simulink model "PSO_ZVD"  (R2021a)
settings: Solver=VariableStepAuto  StartTime=0.0  StopTime=20  RelTol=1e-3
InitFcn:
  | ml=2;
  | 
  | mc=0.5;
  | M2=0.5;
  | 
  | mt=5;
  | g=9.81;
  | l_ref=0.1;
  | l_ini=1;
  | l=l_ini;
  | x_ref=1;
  | n1=5;n2=1;
  | 
  | %ADRC' s parameter caculation
  | %b0 = (ml+mc)/(mc*ml +mc*mt+ml*mt); %Hieu
  | b0=(ml+mc)/(mt*mc+2*ml*mc+mt*ml+ml^2+mc^2); %Enhanced-coupling
  | k_ESO = 100;
  | T_set  = 6;
  | 
  | s_cl = -5.85/T_set;
  | Kp   = s_cl^2;
  | Kd   = -2*s_cl;
  | 
  | s_ESO = k_ESO*s_cl;
  | l1        = -3*s_ESO;
  | l2        = 3*( s_ESO)^2;
  | l3        = -(s_ESO)^3;
  | 
  | %b1 = (mt+mc)/(mc*ml +mc*mt+ml*mt);
  | b1=1/(ml+mc);
  | k_ESO1 =100;
  | T_set1  = 3;
  | s_cl1 = -5.85/T_set1;
  | Kp1   = s_cl1^2;
  | Kd1   = -2*s_cl1;
  | 
  | s_ESO1 = k_ESO1*s_cl1;
  | l11        = -3*s_ESO1;
  | l21        = 3*( s_ESO1)^2;
  | l31        = -(s_ESO1)^3;
  | 
  | 
  | L1=l_ini;
  | %L2=0.5;
  | L2=0.1;
  | m1=2;
  | m2=mc;
  | m=5;
  | %Bo input shaping
  | alpha = (1/L1 + 1/L2)*(m1+M2)/m1;
  | beta = (((m1+M2)/m1)^2)*((1/L1 + 1/L2)^2) - 4*(m1+M2)/(m1*L1*L2);
  | w1 = sqrt(g*(alpha - sqrt(beta))/2);
  | w2 = sqrt(g*(alpha + sqrt(beta))/2);
  | damping_ratio = 0;
  | wd1 = w1*sqrt(1-damping_ratio^2);
  | wd2 = w2*sqrt(1-damping_ratio^2);
  | k = exp(damping_ratio*pi/sqrt(1-damping_ratio^2));
  | 
  | %ZVD1
  | t1_ZVD_1=pi/wd1;
  | ... (+27 lines)
values from neighbouring files (symbols this model uses):
  particle = repmat(empty_particle, nPop, 1)    [PSO16_12.m]    (also in PSO_ZVD.m)
undefined symbols (not defined in the file or in its folder): i, li, xi
libraries: neural x101, simulink_extras x13, simulink x3
(part 3 of 34)

== system PSO_ZVD/RBF_ET4_m=5_m1=2/ADRC 6 ==
  ref : Inport
  x : Inport  Port=2
  Gain : Gain  Gain=Kp1
  Gain1 : Gain  Gain=Kd1
  Gain2 : Gain  Gain=1/b1
  Observer : Subsystem
  Sum : Sum  Inputs=|+-
  Sum3 : Sum  Inputs=|+-
  Sum4 : Sum  Inputs=|+-
  u : Outport
  wires:
  Sum4/1 -> Gain2/1
  Sum/1 -> Gain/1
  Gain2/1 -> u/1, Observer/1(u)
  x/1 -> Observer/2(x)
  Sum3/1 -> Sum4/1
  Observer/2(x2) -> Gain1/1
  Gain1/1 -> Sum3/2
  Gain/1 -> Sum3/1
  ref/1 -> Sum/1
  Observer/1(x3) -> Sum4/2
  Observer/3(x1) -> Sum/2

== system PSO_ZVD/RBF_ET4_m=5_m1=2/ADRC 7 ==
  ref : Inport
  x : Inport  Port=2
  Gain : Gain  Gain=Kp
  Gain1 : Gain  Gain=Kd
  Gain2 : Gain  Gain=1/b0
  Observer : Subsystem
  Sum : Sum  Inputs=|+-
  Sum3 : Sum  Inputs=|+-
  Sum4 : Sum  Inputs=|+-
  u : Outport
  wires:
  Sum4/1 -> Gain2/1
  Sum/1 -> Gain/1
  Gain2/1 -> u/1, Observer/1(u)
  x/1 -> Observer/2(x)
  Sum3/1 -> Sum4/1
  Observer/2(x2) -> Gain1/1
  Gain1/1 -> Sum3/2
  Gain/1 -> Sum3/1
  ref/1 -> Sum/1
  Observer/1(x3) -> Sum4/2
  Observer/3(x1) -> Sum/2

== system PSO_ZVD/RBF_ET4_m=5_m1=2/ADRC 8 ==
  ref : Inport
  x : Inport  Port=2
  Gain : Gain  Gain=Kp1
  Gain1 : Gain  Gain=Kd1
  Gain2 : Gain  Gain=1/b1
  Observer : Subsystem
  Sum : Sum  Inputs=|+-
  Sum3 : Sum  Inputs=|+-
  Sum4 : Sum  Inputs=|+-
  u : Outport
  wires:
  Sum4/1 -> Gain2/1
  Sum/1 -> Gain/1
  Gain2/1 -> u/1, Observer/1(u)
  x/1 -> Observer/2(x)
  Sum3/1 -> Sum4/1
  Observer/2(x2) -> Gain1/1
  Gain1/1 -> Sum3/2
  Gain/1 -> Sum3/1
  ref/1 -> Sum/1
  Observer/1(x3) -> Sum4/2
  Observer/3(x1) -> Sum/2

== system PSO_ZVD/RBF_ET4_m=5_m1=2/ADRC 9 ==
  ref : Inport
  x : Inport  Port=2
  Gain : Gain  Gain=Kp
  Gain1 : Gain  Gain=Kd
  Gain2 : Gain  Gain=1/b0
  Observer : Subsystem
  Sum : Sum  Inputs=|+-
  Sum3 : Sum  Inputs=|+-
  Sum4 : Sum  Inputs=|+-
  u : Outport
  wires:
  Sum4/1 -> Gain2/1
  Sum/1 -> Gain/1
  Gain2/1 -> u/1, Observer/1(u)
  x/1 -> Observer/2(x)
  Sum3/1 -> Sum4/1
  Observer/2(x2) -> Gain1/1
  Gain1/1 -> Sum3/2
  Gain/1 -> Sum3/1
  ref/1 -> Sum/1
  Observer/1(x3) -> Sum4/2
  Observer/3(x1) -> Sum/2

== system PSO_ZVD/RBF_ET4_m=5_m1=2/ETM1 ==
  In1 : Inport
  Gain : Gain  Gain=A1_etm4_2
  Gain1 : Gain  Gain=A2_etm4_2
  Gain2 : Gain  Gain=A3_etm4_2
  Gain3 : Gain  Gain=A4_etm4_2
  Sum : Sum  Inputs=++++
  Transport Delay : TransportDelay  DelayTime=t1_etm4_2
  Transport Delay1 : TransportDelay  DelayTime=t2_etm4_2
  Transport Delay2 : TransportDelay  DelayTime=t3_etm4_2
  ref : Outport
  wires:
  In1/1 -> Gain1/1, Gain3/1, Gain2/1, Gain/1
  Gain1/1 -> Transport Delay/1
  Transport Delay/1 -> Sum/2
  Sum/1 -> ref/1
  Gain2/1 -> Transport Delay1/1
  Gain/1 -> Sum/1
  Transport Delay1/1 -> Sum/3
  Gain3/1 -> Transport Delay2/1
  Transport Delay2/1 -> Sum/4

== system PSO_ZVD/RBF_ET4_m=5_m1=2/ETM2 ==
  ref_ETm4 : Inport
  ETM1 : Subsystem
  ETM4 : Subsystem
  ref1 : Scope
  ref2 : Scope
  ref3 : Scope
  ref_ETM4 : Outport
  wires:
  ETM1/1(Out1) -> ref2/1, ETM4/1(In1)  "ref_ZV"
  ETM4/1(Out1) -> ref3/1, ref_ETM4/1  "ref_ZV"
  ref_ETm4/1 -> ref1/1, ETM1/1(In1)

== system PSO_ZVD/RBF_ET4_m=5_m1=2/ETM3 ==
  In1 : Inport
  Gain : Gain  Gain=A1_etm4_1
  Gain1 : Gain  Gain=A2_etm4_1
  Gain2 : Gain  Gain=A3_etm4_1
  Gain3 : Gain  Gain=A4_etm4_1
  Sum : Sum  Inputs=++++
  Transport Delay : TransportDelay  DelayTime=t1_etm4_1
  Transport Delay1 : TransportDelay  DelayTime=t2_etm4_1
  Transport Delay2 : TransportDelay  DelayTime=t3_etm4_1
  ref : Outport
  wires:
  In1/1 -> Gain1/1, Gain3/1, Gain2/1, Gain/1
  Gain1/1 -> Transport Delay/1
  Transport Delay/1 -> Sum/2
  Sum/1 -> ref/1
  Gain2/1 -> Transport Delay1/1
  Gain/1 -> Sum/1
  Transport Delay1/1 -> Sum/3
  Gain3/1 -> Transport Delay2/1
  Transport Delay2/1 -> Sum/4

== system PSO_ZVD/RBF_ET4_m=5_m1=2/ETM4 ==
  In1 : Inport
  Gain : Gain  Gain=A1_etm4_2
  Gain1 : Gain  Gain=A2_etm4_2
  Gain2 : Gain  Gain=A3_etm4_2
  Gain3 : Gain  Gain=A4_etm4_2
  Sum : Sum  Inputs=++++
  Transport Delay : TransportDelay  DelayTime=t1_etm4_2
  Transport Delay1 : TransportDelay  DelayTime=t2_etm4_2
  Transport Delay2 : TransportDelay  DelayTime=t3_etm4_2
  ref : Outport
  wires:
  In1/1 -> Gain1/1, Gain3/1, Gain2/1, Gain/1
  Gain1/1 -> Transport Delay/1
  Transport Delay/1 -> Sum/2
  Sum/1 -> ref/1
  Gain2/1 -> Transport Delay1/1
  Gain/1 -> Sum/1
  Transport Delay1/1 -> Sum/3
  Gain3/1 -> Transport Delay2/1
  Transport Delay2/1 -> Sum/4

== system PSO_ZVD/RBF_ET4_m=5_m1=2/PSO-ETM1 ==
  In1 : Inport
  Input : Inport  Port=2
  Input1 : Inport  Port=3
  Input2 : Inport  Port=4
  Gain : Gain  Gain=0.1667
  Gain1 : Gain  Gain=0.3333
  Gain2 : Gain  Gain=0.3333
  Gain3 : Gain  Gain=0.1667
  Sum : Sum  Inputs=++++
  Variable Transport Delay : VariableTransportDelay  VariableDelayType=Variable transport delay  MaximumDelay=10
  Variable Transport Delay1 : VariableTransportDelay  VariableDelayType=Variable transport delay  MaximumDelay=10
  Variable Transport Delay2 : VariableTransportDelay  VariableDelayType=Variable transport delay  MaximumDelay=10
  Out1 : Outport
  wires:
  In1/1 -> Gain1/1, Gain3/1, Gain2/1, Gain/1
  Gain1/1 -> Variable Transport Delay/1
  Variable Transport Delay/1 -> Sum/2
  Sum/1 -> Out1/1
  Gain2/1 -> Variable Transport Delay1/1
  Gain/1 -> Sum/1
  Variable Transport Delay1/1 -> Sum/3
  Gain3/1 -> Variable Transport Delay2/1
  Variable Transport Delay2/1 -> Sum/4
  Input/1 -> Variable Transport Delay/2
  Input1/1 -> Variable Transport Delay1/2
  Input2/1 -> Variable Transport Delay2/2

== system PSO_ZVD/RBF_ET4_m=5_m1=2/PSO-ETM3 ==
  In1 : Inport
  Input : Inport  Port=2
  Input1 : Inport  Port=3
  Input2 : Inport  Port=4
  Gain : Gain  Gain=0.1667
  Gain1 : Gain  Gain=0.3333
  Gain2 : Gain  Gain=0.3333
  Gain3 : Gain  Gain=0.1667
  Sum : Sum  Inputs=++++
  Variable Transport Delay : VariableTransportDelay  VariableDelayType=Variable transport delay  MaximumDelay=10
  Variable Transport Delay1 : VariableTransportDelay  VariableDelayType=Variable transport delay  MaximumDelay=10
  Variable Transport Delay2 : VariableTransportDelay  VariableDelayType=Variable transport delay  MaximumDelay=10
  ref : Outport
  wires:
  In1/1 -> Gain1/1, Gain3/1, Gain2/1, Gain/1
  Gain1/1 -> Variable Transport Delay/1
  Variable Transport Delay/1 -> Sum/2
  Sum/1 -> ref/1
  Gain2/1 -> Variable Transport Delay1/1
  Gain/1 -> Sum/1
  Variable Transport Delay1/1 -> Sum/3
  Gain3/1 -> Variable Transport Delay2/1
  Variable Transport Delay2/1 -> Sum/4
  Input/1 -> Variable Transport Delay/2
  Input1/1 -> Variable Transport Delay1/2
  Input2/1 -> Variable Transport Delay2/2

== system PSO_ZVD/RBF_ET4_m=5_m1=2/PSO-ETM4 ==
  In1 : Inport
  Input : Inport  Port=2
  Input1 : Inport  Port=3
  Input2 : Inport  Port=4
  Gain : Gain  Gain=0.1667
  Gain1 : Gain  Gain=0.3333
  Gain2 : Gain  Gain=0.3333
  Gain3 : Gain  Gain=0.1667
  Sum : Sum  Inputs=++++
  Variable Transport Delay : VariableTransportDelay  VariableDelayType=Variable transport delay  MaximumDelay=10
  Variable Transport Delay1 : VariableTransportDelay  VariableDelayType=Variable transport delay  MaximumDelay=10
  Variable Transport Delay2 : VariableTransportDelay  VariableDelayType=Variable transport delay  MaximumDelay=10
  Out1 : Outport
  wires:
  In1/1 -> Gain1/1, Gain3/1, Gain2/1, Gain/1
  Gain1/1 -> Variable Transport Delay/1
  Variable Transport Delay/1 -> Sum/2
  Sum/1 -> Out1/1
  Gain2/1 -> Variable Transport Delay1/1
  Gain/1 -> Sum/1
  Variable Transport Delay1/1 -> Sum/3
  Gain3/1 -> Variable Transport Delay2/1
  Variable Transport Delay2/1 -> Sum/4
  Input/1 -> Variable Transport Delay/2
  Input1/1 -> Variable Transport Delay1/2
  Input2/1 -> Variable Transport Delay2/2

== system PSO_ZVD/RBF_ET4_m=5_m1=2/PSO-ETM5 ==
  In1 : Inport
  Input : Inport  Port=2
  Input1 : Inport  Port=3
  Input2 : Inport  Port=4
  Gain : Gain  Gain=0.1667
  Gain1 : Gain  Gain=0.3333
  Gain2 : Gain  Gain=0.3333
  Gain3 : Gain  Gain=0.1667
  Sum : Sum  Inputs=++++
  Variable Transport Delay : VariableTransportDelay  VariableDelayType=Variable transport delay  MaximumDelay=10
  Variable Transport Delay1 : VariableTransportDelay  VariableDelayType=Variable transport delay  MaximumDelay=10
  Variable Transport Delay2 : VariableTransportDelay  VariableDelayType=Variable transport delay  MaximumDelay=10
  Out1 : Outport
  wires:
  In1/1 -> Gain1/1, Gain3/1, Gain2/1, Gain/1
  Gain1/1 -> Variable Transport Delay/1
  Variable Transport Delay/1 -> Sum/2
  Sum/1 -> Out1/1
  Gain2/1 -> Variable Transport Delay1/1
  Gain/1 -> Sum/1
  Variable Transport Delay1/1 -> Sum/3
  Gain3/1 -> Variable Transport Delay2/1
  Variable Transport Delay2/1 -> Sum/4
  Input/1 -> Variable Transport Delay/2
  Input1/1 -> Variable Transport Delay1/2
  Input2/1 -> Variable Transport Delay2/2

== system PSO_ZVD/RBF_ET4_m=5_m1=2/PSO-ETM6 ==
  In1 : Inport
  Input : Inport  Port=2
  Input1 : Inport  Port=3
  Input2 : Inport  Port=4
  Gain : Gain  Gain=0.1667
  Gain1 : Gain  Gain=0.3333
  Gain2 : Gain  Gain=0.3333
  Gain3 : Gain  Gain=0.1667
  Sum : Sum  Inputs=++++
  Variable Transport Delay : VariableTransportDelay  VariableDelayType=Variable transport delay  MaximumDelay=10
  Variable Transport Delay1 : VariableTransportDelay  VariableDelayType=Variable transport delay  MaximumDelay=10
  Variable Transport Delay2 : VariableTransportDelay  VariableDelayType=Variable transport delay  MaximumDelay=10
  ref : Outport
  wires:
  In1/1 -> Gain1/1, Gain3/1, Gain2/1, Gain/1
  Gain1/1 -> Variable Transport Delay/1
  Variable Transport Delay/1 -> Sum/2
  Sum/1 -> ref/1
  Gain2/1 -> Variable Transport Delay1/1
  Gain/1 -> Sum/1
  Variable Transport Delay1/1 -> Sum/3
  Gain3/1 -> Variable Transport Delay2/1
  Variable Transport Delay2/1 -> Sum/4
  Input/1 -> Variable Transport Delay/2
  Input1/1 -> Variable Transport Delay1/2
  Input2/1 -> Variable Transport Delay2/2

== system PSO_ZVD/RBF_ET4_m=5_m1=2/enhanced1 ==
  Fx : Inport
  Fl : Inport  Port=2
  Add : Sum
  Constant : Constant  Value=-(m1+m2)*g
  Constant1 : Constant  Value=mc
  Crane : MATLAB Function  TreatAsAtomicUnit=on
  Integrator{,1,3,5..7} (6 alike) : Integrator
  Integrator2 : Integrator  InitialCondition=l
  Integrator4 : Integrator  InitialCondition=10*pi/180
  Scope{1..5} (5 alike) : Scope
  x : Outport
  l : Outport  Port=2
  the1 : Outport  Port=3
  the2 : Outport  Port=4
  wires:
  Integrator5/1 -> [x6]
  Integrator2/1 -> Scope4/1, l/1, [x3]
  Integrator1/1 -> [x2]
  Integrator/1 -> x/1, [x1]
  Integrator3/1 -> [x4]
  Add/1 -> Crane/9(Fl), Scope1/1
  Integrator6/1 -> Scope2/1, the2/1, [x7]
  Integrator7/1 -> [x8]
  Crane/1(dx1) -> Integrator/1
  Crane/2(dx2) -> Integrator1/1
  Crane/3(dx3) -> Integrator2/1
  Crane/4(dx4) -> Integrator3/1
  Crane/5(dx5) -> Integrator4/1
  Crane/6(dx6) -> Integrator5/1
  Crane/7(dx7) -> Integrator6/1
  Crane/8(dx8) -> Integrator7/1
  Fx/1 -> Crane/8(Fx)
  Constant1/1 -> Crane/10(m2)
  [x2] -> Crane/1(d1x)
  [x3] -> Crane/2(l1)
  [x4] -> Crane/3(d1l1)
  [x5] -> Crane/4(the1)
  [x6] -> Crane/5(d1the1)
  [x7] -> Crane/6(the2)
  [x8] -> Crane/7(d1the2)
  Integrator4/1 -> Scope3/1, the1/1, [x5]
  Fl/1 -> Add/2
  [x1] -> Scope5/1
  Constant/1 -> Add/1

== system PSO_ZVD/RBF_ET4_m=5_m1=2/enhanced2 ==
  Fx : Inport
  Fl : Inport  Port=2
  Add : Sum
  Constant : Constant  Value=-(m1+m2)*g
  Constant1 : Constant  Value=mc
  Crane : MATLAB Function  TreatAsAtomicUnit=on
  Integrator{,1,3,5..7} (6 alike) : Integrator
  Integrator2 : Integrator  InitialCondition=l
  Integrator4 : Integrator  InitialCondition=10*pi/180
  Scope{1..5} (5 alike) : Scope
  x : Outport
  l : Outport  Port=2
  the1 : Outport  Port=3
  the2 : Outport  Port=4
  wires:
  Integrator5/1 -> [x6]
  Integrator2/1 -> Scope4/1, l/1, [x3]
  Integrator1/1 -> [x2]
  Integrator/1 -> x/1, [x1]
  Integrator3/1 -> [x4]
  Add/1 -> Crane/9(Fl), Scope1/1
  Integrator6/1 -> Scope2/1, the2/1, [x7]
  Integrator7/1 -> [x8]
  Crane/1(dx1) -> Integrator/1
  Crane/2(dx2) -> Integrator1/1
  Crane/3(dx3) -> Integrator2/1
  Crane/4(dx4) -> Integrator3/1
  Crane/5(dx5) -> Integrator4/1
  Crane/6(dx6) -> Integrator5/1
  Crane/7(dx7) -> Integrator6/1
  Crane/8(dx8) -> Integrator7/1
  Fx/1 -> Crane/8(Fx)
  Constant1/1 -> Crane/10(m2)
  [x2] -> Crane/1(d1x)
  [x3] -> Crane/2(l1)
  [x4] -> Crane/3(d1l1)
  [x5] -> Crane/4(the1)
  [x6] -> Crane/5(d1the1)
  [x7] -> Crane/6(the2)
  [x8] -> Crane/7(d1the2)
  Integrator4/1 -> Scope3/1, the1/1, [x5]
  Fl/1 -> Add/2
  [x1] -> Scope5/1
  Constant/1 -> Add/1

== system PSO_ZVD/RBF_ET4_m=5_m1=2/enhanced3 ==
  Fx : Inport
  Fl : Inport  Port=2
  Add : Sum
  Constant : Constant  Value=-(m1+m2)*g
  Constant1 : Constant  Value=mc
  Crane : MATLAB Function  TreatAsAtomicUnit=on
  Integrator{,1,3,5..7} (6 alike) : Integrator
  Integrator2 : Integrator  InitialCondition=l
  Integrator4 : Integrator  InitialCondition=10*pi/180
  Scope{1..5} (5 alike) : Scope
  x : Outport
  l : Outport  Port=2
  the1 : Outport  Port=3
  the2 : Outport  Port=4
  wires:
  Integrator5/1 -> [x6]
  Integrator2/1 -> Scope4/1, l/1, [x3]
  Integrator1/1 -> [x2]
  Integrator/1 -> x/1, [x1]
  Integrator3/1 -> [x4]
  Add/1 -> Crane/9(Fl), Scope1/1
  Integrator6/1 -> Scope2/1, the2/1, [x7]
  Integrator7/1 -> [x8]
  Crane/1(dx1) -> Integrator/1
  Crane/2(dx2) -> Integrator1/1
  Crane/3(dx3) -> Integrator2/1
  Crane/4(dx4) -> Integrator3/1
  Crane/5(dx5) -> Integrator4/1
  Crane/6(dx6) -> Integrator5/1
  Crane/7(dx7) -> Integrator6/1
  Crane/8(dx8) -> Integrator7/1
  Fx/1 -> Crane/8(Fx)
  Constant1/1 -> Crane/10(m2)
  [x2] -> Crane/1(d1x)
  [x3] -> Crane/2(l1)
  [x4] -> Crane/3(d1l1)
  [x5] -> Crane/4(the1)
  [x6] -> Crane/5(d1the1)
  [x7] -> Crane/6(the2)
  [x8] -> Crane/7(d1the2)
  Integrator4/1 -> Scope3/1, the1/1, [x5]
  Fl/1 -> Add/2
  [x1] -> Scope5/1
  Constant/1 -> Add/1

== system PSO_ZVD/RBF_ET4_m=5_m1=2/enhanced4 ==
  Fx : Inport
  Fl : Inport  Port=2
  Add : Sum
  Constant : Constant  Value=-(m1+m2)*g
  Constant1 : Constant  Value=mc
  Crane : MATLAB Function  TreatAsAtomicUnit=on
  Integrator{,1,3,5..7} (6 alike) : Integrator
  Integrator2 : Integrator  InitialCondition=l
  Integrator4 : Integrator  InitialCondition=10*pi/180
  Scope{1..5} (5 alike) : Scope
  x : Outport
  l : Outport  Port=2
  the1 : Outport  Port=3
  the2 : Outport  Port=4
  wires:
  Integrator5/1 -> [x6]
  Integrator2/1 -> Scope4/1, l/1, [x3]
  Integrator1/1 -> [x2]
  Integrator/1 -> x/1, [x1]
  Integrator3/1 -> [x4]
  Add/1 -> Crane/9(Fl), Scope1/1
  Integrator6/1 -> Scope2/1, the2/1, [x7]
  Integrator7/1 -> [x8]
  Crane/1(dx1) -> Integrator/1
  Crane/2(dx2) -> Integrator1/1
  Crane/3(dx3) -> Integrator2/1
  Crane/4(dx4) -> Integrator3/1
  Crane/5(dx5) -> Integrator4/1
  Crane/6(dx6) -> Integrator5/1
  Crane/7(dx7) -> Integrator6/1
  Crane/8(dx8) -> Integrator7/1
  Fx/1 -> Crane/8(Fx)
  Constant1/1 -> Crane/10(m2)
  [x2] -> Crane/1(d1x)
  [x3] -> Crane/2(l1)
  [x4] -> Crane/3(d1l1)
  [x5] -> Crane/4(the1)
  [x6] -> Crane/5(d1the1)
  [x7] -> Crane/6(the2)
  [x8] -> Crane/7(d1the2)
  Integrator4/1 -> Scope3/1, the1/1, [x5]
  Fl/1 -> Add/2
  [x1] -> Scope5/1
  Constant/1 -> Add/1

== system PSO_ZVD/RBF_ET4_m=5_m1=2/enhanced5 ==
  Fx : Inport
  Fl : Inport  Port=2
  Add : Sum
  Constant : Constant  Value=-(m1+m2)*g
  Constant1 : Constant  Value=mc
  Crane : MATLAB Function  TreatAsAtomicUnit=on
  Integrator{,1,3,5..7} (6 alike) : Integrator
  Integrator2 : Integrator  InitialCondition=l
  Integrator4 : Integrator  InitialCondition=10*pi/180
  Scope{1..5} (5 alike) : Scope
  x : Outport
  l : Outport  Port=2
  the1 : Outport  Port=3
  the2 : Outport  Port=4
  wires:
  Integrator5/1 -> [x6]
  Integrator2/1 -> Scope4/1, l/1, [x3]
  Integrator1/1 -> [x2]
  Integrator/1 -> x/1, [x1]
  Integrator3/1 -> [x4]
  Add/1 -> Crane/9(Fl), Scope1/1
  Integrator6/1 -> Scope2/1, the2/1, [x7]
  Integrator7/1 -> [x8]
  Crane/1(dx1) -> Integrator/1
  Crane/2(dx2) -> Integrator1/1
  Crane/3(dx3) -> Integrator2/1
  Crane/4(dx4) -> Integrator3/1
  Crane/5(dx5) -> Integrator4/1
  Crane/6(dx6) -> Integrator5/1
  Crane/7(dx7) -> Integrator6/1
  Crane/8(dx8) -> Integrator7/1
  Fx/1 -> Crane/8(Fx)
  Constant1/1 -> Crane/10(m2)
  [x2] -> Crane/1(d1x)
  [x3] -> Crane/2(l1)
  [x4] -> Crane/3(d1l1)
  [x5] -> Crane/4(the1)
  [x6] -> Crane/5(d1the1)
  [x7] -> Crane/6(the2)
  [x8] -> Crane/7(d1the2)
  Integrator4/1 -> Scope3/1, the1/1, [x5]
  Fl/1 -> Add/2
  [x1] -> Scope5/1
  Constant/1 -> Add/1

== system PSO_ZVD/RBF_ET4_m=5_m1=2/enhanced6 ==
  Fx : Inport
  Fl : Inport  Port=2
  Add : Sum
  Constant : Constant  Value=-(m1+m2)*g
  Constant1 : Constant  Value=mc
  Crane : MATLAB Function  TreatAsAtomicUnit=on
  Integrator{,1,3,5..7} (6 alike) : Integrator
  Integrator2 : Integrator  InitialCondition=l
  Integrator4 : Integrator  InitialCondition=10*pi/180
  Scope{1..5} (5 alike) : Scope
  x : Outport
  l : Outport  Port=2
  the1 : Outport  Port=3
  the2 : Outport  Port=4
  wires:
  Integrator5/1 -> [x6]
  Integrator2/1 -> Scope4/1, l/1, [x3]
  Integrator1/1 -> [x2]
  Integrator/1 -> x/1, [x1]
  Integrator3/1 -> [x4]
  Add/1 -> Crane/9(Fl), Scope1/1
  Integrator6/1 -> Scope2/1, the2/1, [x7]
  Integrator7/1 -> [x8]
  Crane/1(dx1) -> Integrator/1
  Crane/2(dx2) -> Integrator1/1
  Crane/3(dx3) -> Integrator2/1
  Crane/4(dx4) -> Integrator3/1
  Crane/5(dx5) -> Integrator4/1
  Crane/6(dx6) -> Integrator5/1
  Crane/7(dx7) -> Integrator6/1
  Crane/8(dx8) -> Integrator7/1
  Fx/1 -> Crane/8(Fx)
  Constant1/1 -> Crane/10(m2)
  [x2] -> Crane/1(d1x)
  [x3] -> Crane/2(l1)
  [x4] -> Crane/3(d1l1)
  [x5] -> Crane/4(the1)
  [x6] -> Crane/5(d1the1)
  [x7] -> Crane/6(the2)
  [x8] -> Crane/7(d1the2)
  Integrator4/1 -> Scope3/1, the1/1, [x5]
  Fl/1 -> Add/2
  [x1] -> Scope5/1
  Constant/1 -> Add/1

== system PSO_ZVD/RBF_ET4_m=5_m1=2/m=5; m1=2_LT ==
  Input : Inport  PortDimensions=2
      mask Display: e = 0.06;c1 = [120 230 180]/255;c2 = ([120 230 180]+0)/(256+128);c3 = ([120 230 180]+128)/(256+128);patch([0 1 1 0],[0 0 1 1],c1);patch([0 1 1 1-e 1-e 0+e],[0 0 1 1-e 0+e 0+e],c2);patch([0 0 1 1-e 0+e 0+e],[0 1 1 1-e 1-e 0+e],c3);plot([0 1 1 0 0],[0 0 1 1 0]);
  Layer 1 : Subsystem
      mask Display: e = 0.06;c1 = [120 150 230]/255;c2 = ([120 150 230]+0)/383;c3 = ([120 150 230]+128)/383;patch([0 1 1 0],[0 0 1 1],c1);patch([0 1 1 1-e 1-e 0+e],[0 0 1 1-e 0+e 0+e],c2);patch([0 0 1 1-e 0+e 0+e],[0 1 1 1-e 1-e 0+e],c3);plot([0 1 1 0 0],[0 0 1 1 0]);
  Layer 2 : Subsystem
      mask Display: e = 0.06;c1 = [120 150 230]/255;c2 = ([120 150 230]+0)/383;c3 = ([120 150 230]+128)/383;patch([0 1 1 0],[0 0 1 1],c1);patch([0 1 1 1-e 1-e 0+e],[0 0 1 1-e 0+e 0+e],c2);patch([0 0 1 1-e 0+e 0+e],[0 1 1 1-e 1-e 0+e],c3);plot([0 1 1 0 0],[0 0 1 1 0]);
  Process Input 1 : Subsystem
      mask Display: e = 0.06;c1 = [120 150 230]/255;c2 = ([120 150 230]+0)/383;c3 = ([120 150 230]+128)/383;patch([0 1 1 0],[0 0 1 1],c1);patch([0 1 1 1-e 1-e 0+e],[0 0 1 1-e 0+e 0+e],c2);patch([0 0 1 1-e 0+e 0+e],[0 1 1 1-e 1-e 0+e],c3);plot([0 1 1 0 0],[0 0 1 1 0]);
  Process Output 1 : Subsystem
      mask Display: e = 0.06;c1 = [120 150 230]/255;c2 = ([120 150 230]+0)/383;c3 = ([120 150 230]+128)/383;patch([0 1 1 0],[0 0 1 1],c1);patch([0 1 1 1-e 1-e 0+e],[0 0 1 1-e 0+e 0+e],c2);patch([0 0 1 1-e 0+e 0+e],[0 1 1 1-e 1-e 0+e],c3);plot([0 1 1 0 0],[0 0 1 1 0]);
  Output : Outport  InitialOutput=[0;0;0]
      mask Display: e = 0.06;c1 = [120 230 180]/255;c2 = ([120 230 180]+0)/(256+128);c3 = ([120 230 180]+128)/(256+128);patch([0 1 1 0],[0 0 1 1],c1);patch([0 1 1 1-e 1-e 0+e],[0 0 1 1-e 0+e 0+e],c2);patch([0 0 1 1-e 0+e 0+e],[0 1 1 1-e 1-e 0+e],c3);plot([0 1 1 0 0],[0 0 1 1 0]);
  wires:
  Input/1 -> Process Input 1/1(x)
  Process Output 1/1(y) -> Output/1
  Process Input 1/1(p) -> Layer 1/1("p{1}")
  Layer 1/1("a{1}") -> [feedback1]
  [feedback1] -> Layer 2/1("a{1} ")
  Layer 2/1("a{2}") -> Process Output 1/1(a)

== system PSO_ZVD/RBF_ET4_m=5_m1=2/m=5; m1=2_LT-bo 1 ==
  Input : Inport  PortDimensions=2
      mask Display: e = 0.06;c1 = [120 230 180]/255;c2 = ([120 230 180]+0)/(256+128);c3 = ([120 230 180]+128)/(256+128);patch([0 1 1 0],[0 0 1 1],c1);patch([0 1 1 1-e 1-e 0+e],[0 0 1 1-e 0+e 0+e],c2);patch([0 0 1 1-e 0+e 0+e],[0 1 1 1-e 1-e 0+e],c3);plot([0 1 1 0 0],[0 0 1 1 0]);
  Layer 1 : Subsystem
      mask Display: e = 0.06;c1 = [120 150 230]/255;c2 = ([120 150 230]+0)/383;c3 = ([120 150 230]+128)/383;patch([0 1 1 0],[0 0 1 1],c1);patch([0 1 1 1-e 1-e 0+e],[0 0 1 1-e 0+e 0+e],c2);patch([0 0 1 1-e 0+e 0+e],[0 1 1 1-e 1-e 0+e],c3);plot([0 1 1 0 0],[0 0 1 1 0]);
  Layer 2 : Subsystem
      mask Display: e = 0.06;c1 = [120 150 230]/255;c2 = ([120 150 230]+0)/383;c3 = ([120 150 230]+128)/383;patch([0 1 1 0],[0 0 1 1],c1);patch([0 1 1 1-e 1-e 0+e],[0 0 1 1-e 0+e 0+e],c2);patch([0 0 1 1-e 0+e 0+e],[0 1 1 1-e 1-e 0+e],c3);plot([0 1 1 0 0],[0 0 1 1 0]);
  Process Input 1 : Subsystem
      mask Display: e = 0.06;c1 = [120 150 230]/255;c2 = ([120 150 230]+0)/383;c3 = ([120 150 230]+128)/383;patch([0 1 1 0],[0 0 1 1],c1);patch([0 1 1 1-e 1-e 0+e],[0 0 1 1-e 0+e 0+e],c2);patch([0 0 1 1-e 0+e 0+e],[0 1 1 1-e 1-e 0+e],c3);plot([0 1 1 0 0],[0 0 1 1 0]);
  Process Output 1 : Subsystem
      mask Display: e = 0.06;c1 = [120 150 230]/255;c2 = ([120 150 230]+0)/383;c3 = ([120 150 230]+128)/383;patch([0 1 1 0],[0 0 1 1],c1);patch([0 1 1 1-e 1-e 0+e],[0 0 1 1-e 0+e 0+e],c2);patch([0 0 1 1-e 0+e 0+e],[0 1 1 1-e 1-e 0+e],c3);plot([0 1 1 0 0],[0 0 1 1 0]);
  Output : Outport  InitialOutput=[0;0;0]
      mask Display: e = 0.06;c1 = [120 230 180]/255;c2 = ([120 230 180]+0)/(256+128);c3 = ([120 230 180]+128)/(256+128);patch([0 1 1 0],[0 0 1 1],c1);patch([0 1 1 1-e 1-e 0+e],[0 0 1 1-e 0+e 0+e],c2);patch([0 0 1 1-e 0+e 0+e],[0 1 1 1-e 1-e 0+e],c3);plot([0 1 1 0 0],[0 0 1 1 0]);
  wires:
  Input/1 -> Process Input 1/1(x)
  Process Output 1/1(y) -> Output/1
  Process Input 1/1(p) -> Layer 1/1("p{1}")
  Layer 1/1("a{1}") -> [feedback1]
  [feedback1] -> Layer 2/1("a{1} ")
  Layer 2/1("a{2}") -> Process Output 1/1(a)

== system PSO_ZVD/RBF_ET4_m=5_m1=2/m=5; m1=2_LT-bo 2 ==
  Input : Inport  PortDimensions=2
      mask Display: e = 0.06;c1 = [120 230 180]/255;c2 = ([120 230 180]+0)/(256+128);c3 = ([120 230 180]+128)/(256+128);patch([0 1 1 0],[0 0 1 1],c1);patch([0 1 1 1-e 1-e 0+e],[0 0 1 1-e 0+e 0+e],c2);patch([0 0 1 1-e 0+e 0+e],[0 1 1 1-e 1-e 0+e],c3);plot([0 1 1 0 0],[0 0 1 1 0]);
  Layer 1 : Subsystem
      mask Display: e = 0.06;c1 = [120 150 230]/255;c2 = ([120 150 230]+0)/383;c3 = ([120 150 230]+128)/383;patch([0 1 1 0],[0 0 1 1],c1);patch([0 1 1 1-e 1-e 0+e],[0 0 1 1-e 0+e 0+e],c2);patch([0 0 1 1-e 0+e 0+e],[0 1 1 1-e 1-e 0+e],c3);plot([0 1 1 0 0],[0 0 1 1 0]);
  Layer 2 : Subsystem
      mask Display: e = 0.06;c1 = [120 150 230]/255;c2 = ([120 150 230]+0)/383;c3 = ([120 150 230]+128)/383;patch([0 1 1 0],[0 0 1 1],c1);patch([0 1 1 1-e 1-e 0+e],[0 0 1 1-e 0+e 0+e],c2);patch([0 0 1 1-e 0+e 0+e],[0 1 1 1-e 1-e 0+e],c3);plot([0 1 1 0 0],[0 0 1 1 0]);
  Process Input 1 : Subsystem
      mask Display: e = 0.06;c1 = [120 150 230]/255;c2 = ([120 150 230]+0)/383;c3 = ([120 150 230]+128)/383;patch([0 1 1 0],[0 0 1 1],c1);patch([0 1 1 1-e 1-e 0+e],[0 0 1 1-e 0+e 0+e],c2);patch([0 0 1 1-e 0+e 0+e],[0 1 1 1-e 1-e 0+e],c3);plot([0 1 1 0 0],[0 0 1 1 0]);
  Process Output 1 : Subsystem
      mask Display: e = 0.06;c1 = [120 150 230]/255;c2 = ([120 150 230]+0)/383;c3 = ([120 150 230]+128)/383;patch([0 1 1 0],[0 0 1 1],c1);patch([0 1 1 1-e 1-e 0+e],[0 0 1 1-e 0+e 0+e],c2);patch([0 0 1 1-e 0+e 0+e],[0 1 1 1-e 1-e 0+e],c3);plot([0 1 1 0 0],[0 0 1 1 0]);
  Output : Outport  InitialOutput=[0;0;0]
      mask Display: e = 0.06;c1 = [120 230 180]/255;c2 = ([120 230 180]+0)/(256+128);c3 = ([120 230 180]+128)/(256+128);patch([0 1 1 0],[0 0 1 1],c1);patch([0 1 1 1-e 1-e 0+e],[0 0 1 1-e 0+e 0+e],c2);patch([0 0 1 1-e 0+e 0+e],[0 1 1 1-e 1-e 0+e],c3);plot([0 1 1 0 0],[0 0 1 1 0]);
  wires:
  Input/1 -> Process Input 1/1(x)
  Process Output 1/1(y) -> Output/1
  Process Input 1/1(p) -> Layer 1/1("p{1}")
  Layer 1/1("a{1}") -> [feedback1]
  [feedback1] -> Layer 2/1("a{1} ")
  Layer 2/1("a{2}") -> Process Output 1/1(a)

== system PSO_ZVD/RBF_ET4_m=5_m1=2/m=5; m1=2_LT-chi bo 2 ==
  Input : Inport  PortDimensions=2
      mask Display: e = 0.06;c1 = [120 230 180]/255;c2 = ([120 230 180]+0)/(256+128);c3 = ([120 230 180]+128)/(256+128);patch([0 1 1 0],[0 0 1 1],c1);patch([0 1 1 1-e 1-e 0+e],[0 0 1 1-e 0+e 0+e],c2);patch([0 0 1 1-e 0+e 0+e],[0 1 1 1-e 1-e 0+e],c3);plot([0 1 1 0 0],[0 0 1 1 0]);
  Layer 1 : Subsystem
      mask Display: e = 0.06;c1 = [120 150 230]/255;c2 = ([120 150 230]+0)/383;c3 = ([120 150 230]+128)/383;patch([0 1 1 0],[0 0 1 1],c1);patch([0 1 1 1-e 1-e 0+e],[0 0 1 1-e 0+e 0+e],c2);patch([0 0 1 1-e 0+e 0+e],[0 1 1 1-e 1-e 0+e],c3);plot([0 1 1 0 0],[0 0 1 1 0]);
  Layer 2 : Subsystem
      mask Display: e = 0.06;c1 = [120 150 230]/255;c2 = ([120 150 230]+0)/383;c3 = ([120 150 230]+128)/383;patch([0 1 1 0],[0 0 1 1],c1);patch([0 1 1 1-e 1-e 0+e],[0 0 1 1-e 0+e 0+e],c2);patch([0 0 1 1-e 0+e 0+e],[0 1 1 1-e 1-e 0+e],c3);plot([0 1 1 0 0],[0 0 1 1 0]);
  Process Input 1 : Subsystem
      mask Display: e = 0.06;c1 = [120 150 230]/255;c2 = ([120 150 230]+0)/383;c3 = ([120 150 230]+128)/383;patch([0 1 1 0],[0 0 1 1],c1);patch([0 1 1 1-e 1-e 0+e],[0 0 1 1-e 0+e 0+e],c2);patch([0 0 1 1-e 0+e 0+e],[0 1 1 1-e 1-e 0+e],c3);plot([0 1 1 0 0],[0 0 1 1 0]);
  Process Output 1 : Subsystem
      mask Display: e = 0.06;c1 = [120 150 230]/255;c2 = ([120 150 230]+0)/383;c3 = ([120 150 230]+128)/383;patch([0 1 1 0],[0 0 1 1],c1);patch([0 1 1 1-e 1-e 0+e],[0 0 1 1-e 0+e 0+e],c2);patch([0 0 1 1-e 0+e 0+e],[0 1 1 1-e 1-e 0+e],c3);plot([0 1 1 0 0],[0 0 1 1 0]);
  Output : Outport  InitialOutput=[0;0;0]
      mask Display: e = 0.06;c1 = [120 230 180]/255;c2 = ([120 230 180]+0)/(256+128);c3 = ([120 230 180]+128)/(256+128);patch([0 1 1 0],[0 0 1 1],c1);patch([0 1 1 1-e 1-e 0+e],[0 0 1 1-e 0+e 0+e],c2);patch([0 0 1 1-e 0+e 0+e],[0 1 1 1-e 1-e 0+e],c3);plot([0 1 1 0 0],[0 0 1 1 0]);
  wires:
  Input/1 -> Process Input 1/1(x)
  Process Output 1/1(y) -> Output/1
  Process Input 1/1(p) -> Layer 1/1("p{1}")
  Layer 1/1("a{1}") -> [feedback1]
  [feedback1] -> Layer 2/1("a{1} ")
  Layer 2/1("a{2}") -> Process Output 1/1(a)

== system PSO_ZVD/RBF_ET4_m=5_m1=2/m=5; m1=2_PSO ==
  Input : Inport  PortDimensions=2
      mask Display: e = 0.06;c1 = [120 230 180]/255;c2 = ([120 230 180]+0)/(256+128);c3 = ([120 230 180]+128)/(256+128);patch([0 1 1 0],[0 0 1 1],c1);patch([0 1 1 1-e 1-e 0+e],[0 0 1 1-e 0+e 0+e],c2);patch([0 0 1 1-e 0+e 0+e],[0 1 1 1-e 1-e 0+e],c3);plot([0 1 1 0 0],[0 0 1 1 0]);
  Layer 1 : Subsystem
      mask Display: e = 0.06;c1 = [120 150 230]/255;c2 = ([120 150 230]+0)/383;c3 = ([120 150 230]+128)/383;patch([0 1 1 0],[0 0 1 1],c1);patch([0 1 1 1-e 1-e 0+e],[0 0 1 1-e 0+e 0+e],c2);patch([0 0 1 1-e 0+e 0+e],[0 1 1 1-e 1-e 0+e],c3);plot([0 1 1 0 0],[0 0 1 1 0]);
  Layer 2 : Subsystem
      mask Display: e = 0.06;c1 = [120 150 230]/255;c2 = ([120 150 230]+0)/383;c3 = ([120 150 230]+128)/383;patch([0 1 1 0],[0 0 1 1],c1);patch([0 1 1 1-e 1-e 0+e],[0 0 1 1-e 0+e 0+e],c2);patch([0 0 1 1-e 0+e 0+e],[0 1 1 1-e 1-e 0+e],c3);plot([0 1 1 0 0],[0 0 1 1 0]);
  Process Input 1 : Subsystem
      mask Display: e = 0.06;c1 = [120 150 230]/255;c2 = ([120 150 230]+0)/383;c3 = ([120 150 230]+128)/383;patch([0 1 1 0],[0 0 1 1],c1);patch([0 1 1 1-e 1-e 0+e],[0 0 1 1-e 0+e 0+e],c2);patch([0 0 1 1-e 0+e 0+e],[0 1 1 1-e 1-e 0+e],c3);plot([0 1 1 0 0],[0 0 1 1 0]);
  Process Output 1 : Subsystem
      mask Display: e = 0.06;c1 = [120 150 230]/255;c2 = ([120 150 230]+0)/383;c3 = ([120 150 230]+128)/383;patch([0 1 1 0],[0 0 1 1],c1);patch([0 1 1 1-e 1-e 0+e],[0 0 1 1-e 0+e 0+e],c2);patch([0 0 1 1-e 0+e 0+e],[0 1 1 1-e 1-e 0+e],c3);plot([0 1 1 0 0],[0 0 1 1 0]);
  Output : Outport  InitialOutput=[0;0;0]
      mask Display: e = 0.06;c1 = [120 230 180]/255;c2 = ([120 230 180]+0)/(256+128);c3 = ([120 230 180]+128)/(256+128);patch([0 1 1 0],[0 0 1 1],c1);patch([0 1 1 1-e 1-e 0+e],[0 0 1 1-e 0+e 0+e],c2);patch([0 0 1 1-e 0+e 0+e],[0 1 1 1-e 1-e 0+e],c3);plot([0 1 1 0 0],[0 0 1 1 0]);
  wires:
  Input/1 -> Process Input 1/1(x)
  Process Output 1/1(y) -> Output/1
  Process Input 1/1(p) -> Layer 1/1("p{1}")
  Layer 1/1("a{1}") -> [feedback1]
  [feedback1] -> Layer 2/1("a{1} ")
  Layer 2/1("a{2}") -> Process Output 1/1(a)

== system PSO_ZVD/RBF_ZVD_m=5_m1=1/ADRC 1 ==
  ref : Inport
  x : Inport  Port=2
  Gain : Gain  Gain=Kp
  Gain1 : Gain  Gain=Kd
  Gain2 : Gain  Gain=1/b0
  Observer : Subsystem
  Sum : Sum  Inputs=|+-
  Sum3 : Sum  Inputs=|+-
  Sum4 : Sum  Inputs=|+-
  u : Outport
  wires:
  Sum4/1 -> Gain2/1
  Sum/1 -> Gain/1
  Gain2/1 -> u/1, Observer/1(u)
  x/1 -> Observer/2(x)
  Sum3/1 -> Sum4/1
  Observer/2(x2) -> Gain1/1
  Gain1/1 -> Sum3/2
  Gain/1 -> Sum3/1
  ref/1 -> Sum/1
  Observer/1(x3) -> Sum4/2
  Observer/3(x1) -> Sum/2

== system PSO_ZVD/RBF_ZVD_m=5_m1=1/ADRC 10 ==
  ref : Inport
  x : Inport  Port=2
  Gain : Gain  Gain=Kp
  Gain1 : Gain  Gain=Kd
  Gain2 : Gain  Gain=1/b0
  Observer : Subsystem
  Sum : Sum  Inputs=|+-
  Sum3 : Sum  Inputs=|+-
  Sum4 : Sum  Inputs=|+-
  u : Outport
  wires:
  Sum4/1 -> Gain2/1
  Sum/1 -> Gain/1
  Gain2/1 -> u/1, Observer/1(u)
  x/1 -> Observer/2(x)
  Sum3/1 -> Sum4/1
  Observer/2(x2) -> Gain1/1
  Gain1/1 -> Sum3/2
  Gain/1 -> Sum3/1
  ref/1 -> Sum/1
  Observer/1(x3) -> Sum4/2
  Observer/3(x1) -> Sum/2

== system PSO_ZVD/RBF_ZVD_m=5_m1=1/ADRC 11 ==
  ref : Inport
  x : Inport  Port=2
  Gain : Gain  Gain=Kp1
  Gain1 : Gain  Gain=Kd1
  Gain2 : Gain  Gain=1/b1
  Observer : Subsystem
  Sum : Sum  Inputs=|+-
  Sum3 : Sum  Inputs=|+-
  Sum4 : Sum  Inputs=|+-
  u : Outport
  wires:
  Sum4/1 -> Gain2/1
  Sum/1 -> Gain/1
  Gain2/1 -> u/1, Observer/1(u)
  x/1 -> Observer/2(x)
  Sum3/1 -> Sum4/1
  Observer/2(x2) -> Gain1/1
  Gain1/1 -> Sum3/2
  Gain/1 -> Sum3/1
  ref/1 -> Sum/1
  Observer/1(x3) -> Sum4/2
  Observer/3(x1) -> Sum/2

== system PSO_ZVD/RBF_ZVD_m=5_m1=1/ADRC 12 ==
  ref : Inport
  x : Inport  Port=2
  Gain : Gain  Gain=Kp1
  Gain1 : Gain  Gain=Kd1
  Gain2 : Gain  Gain=1/b1
  Observer : Subsystem
  Sum : Sum  Inputs=|+-
  Sum3 : Sum  Inputs=|+-
  Sum4 : Sum  Inputs=|+-
  u : Outport
  wires:
  Sum4/1 -> Gain2/1
  Sum/1 -> Gain/1
  Gain2/1 -> u/1, Observer/1(u)
  x/1 -> Observer/2(x)
  Sum3/1 -> Sum4/1
  Observer/2(x2) -> Gain1/1
  Gain1/1 -> Sum3/2
  Gain/1 -> Sum3/1
  ref/1 -> Sum/1
  Observer/1(x3) -> Sum4/2
  Observer/3(x1) -> Sum/2

== system PSO_ZVD/RBF_ZVD_m=5_m1=1/ADRC 2 ==
  ref : Inport
  x : Inport  Port=2
  Gain : Gain  Gain=Kp1
  Gain1 : Gain  Gain=Kd1
  Gain2 : Gain  Gain=1/b1
  Observer : Subsystem
  Sum : Sum  Inputs=|+-
  Sum3 : Sum  Inputs=|+-
  Sum4 : Sum  Inputs=|+-
  u : Outport
  wires:
  Sum4/1 -> Gain2/1
  Sum/1 -> Gain/1
  Gain2/1 -> u/1, Observer/1(u)
  x/1 -> Observer/2(x)
  Sum3/1 -> Sum4/1
  Observer/2(x2) -> Gain1/1
  Gain1/1 -> Sum3/2
  Gain/1 -> Sum3/1
  ref/1 -> Sum/1
  Observer/1(x3) -> Sum4/2
  Observer/3(x1) -> Sum/2

== system PSO_ZVD/RBF_ZVD_m=5_m1=1/ADRC 3 ==
  ref : Inport
  x : Inport  Port=2
  Gain : Gain  Gain=Kp
  Gain1 : Gain  Gain=Kd
  Gain2 : Gain  Gain=1/b0
  Observer : Subsystem
  Sum : Sum  Inputs=|+-
  Sum3 : Sum  Inputs=|+-
  Sum4 : Sum  Inputs=|+-
  u : Outport
  wires:
  Sum4/1 -> Gain2/1
  Sum/1 -> Gain/1
  Gain2/1 -> u/1, Observer/1(u)
  x/1 -> Observer/2(x)
  Sum3/1 -> Sum4/1
  Observer/2(x2) -> Gain1/1
  Gain1/1 -> Sum3/2
  Gain/1 -> Sum3/1
  ref/1 -> Sum/1
  Observer/1(x3) -> Sum4/2
  Observer/3(x1) -> Sum/2

== system PSO_ZVD/RBF_ZVD_m=5_m1=1/ADRC 4 ==
  ref : Inport
  x : Inport  Port=2
  Gain : Gain  Gain=Kp1
  Gain1 : Gain  Gain=Kd1
  Gain2 : Gain  Gain=1/b1
  Observer : Subsystem
  Sum : Sum  Inputs=|+-
  Sum3 : Sum  Inputs=|+-
  Sum4 : Sum  Inputs=|+-
  u : Outport
  wires:
  Sum4/1 -> Gain2/1
  Sum/1 -> Gain/1
  Gain2/1 -> u/1, Observer/1(u)
  x/1 -> Observer/2(x)
  Sum3/1 -> Sum4/1
  Observer/2(x2) -> Gain1/1
  Gain1/1 -> Sum3/2
  Gain/1 -> Sum3/1
  ref/1 -> Sum/1
  Observer/1(x3) -> Sum4/2
  Observer/3(x1) -> Sum/2

== system PSO_ZVD/RBF_ZVD_m=5_m1=1/ADRC 5 ==
  ref : Inport
  x : Inport  Port=2
  Gain : Gain  Gain=Kp
  Gain1 : Gain  Gain=Kd
  Gain2 : Gain  Gain=1/b0
  Observer : Subsystem
  Sum : Sum  Inputs=|+-
  Sum3 : Sum  Inputs=|+-
  Sum4 : Sum  Inputs=|+-
  u : Outport
  wires:
  Sum4/1 -> Gain2/1
  Sum/1 -> Gain/1
  Gain2/1 -> u/1, Observer/1(u)
  x/1 -> Observer/2(x)
  Sum3/1 -> Sum4/1
  Observer/2(x2) -> Gain1/1
  Gain1/1 -> Sum3/2
  Gain/1 -> Sum3/1
  ref/1 -> Sum/1
  Observer/1(x3) -> Sum4/2
  Observer/3(x1) -> Sum/2

== system PSO_ZVD/RBF_ZVD_m=5_m1=1/ADRC 6 ==
  ref : Inport
  x : Inport  Port=2
  Gain : Gain  Gain=Kp1
  Gain1 : Gain  Gain=Kd1
  Gain2 : Gain  Gain=1/b1
  Observer : Subsystem
  Sum : Sum  Inputs=|+-
  Sum3 : Sum  Inputs=|+-
  Sum4 : Sum  Inputs=|+-
  u : Outport
  wires:
  Sum4/1 -> Gain2/1
  Sum/1 -> Gain/1
  Gain2/1 -> u/1, Observer/1(u)
  x/1 -> Observer/2(x)
  Sum3/1 -> Sum4/1
  Observer/2(x2) -> Gain1/1
  Gain1/1 -> Sum3/2
  Gain/1 -> Sum3/1
  ref/1 -> Sum/1
  Observer/1(x3) -> Sum4/2
  Observer/3(x1) -> Sum/2

== system PSO_ZVD/RBF_ZVD_m=5_m1=1/ADRC 7 ==
  ref : Inport
  x : Inport  Port=2
  Gain : Gain  Gain=Kp
  Gain1 : Gain  Gain=Kd
  Gain2 : Gain  Gain=1/b0
  Observer : Subsystem
  Sum : Sum  Inputs=|+-
  Sum3 : Sum  Inputs=|+-
  Sum4 : Sum  Inputs=|+-
  u : Outport
  wires:
  Sum4/1 -> Gain2/1
  Sum/1 -> Gain/1
  Gain2/1 -> u/1, Observer/1(u)
  x/1 -> Observer/2(x)
  Sum3/1 -> Sum4/1
  Observer/2(x2) -> Gain1/1
  Gain1/1 -> Sum3/2
  Gain/1 -> Sum3/1
  ref/1 -> Sum/1
  Observer/1(x3) -> Sum4/2
  Observer/3(x1) -> Sum/2

== system PSO_ZVD/RBF_ZVD_m=5_m1=1/ADRC 8 ==
  ref : Inport
  x : Inport  Port=2
  Gain : Gain  Gain=Kp1
  Gain1 : Gain  Gain=Kd1
  Gain2 : Gain  Gain=1/b1
  Observer : Subsystem
  Sum : Sum  Inputs=|+-
  Sum3 : Sum  Inputs=|+-
  Sum4 : Sum  Inputs=|+-
  u : Outport
  wires:
  Sum4/1 -> Gain2/1
  Sum/1 -> Gain/1
  Gain2/1 -> u/1, Observer/1(u)
  x/1 -> Observer/2(x)
  Sum3/1 -> Sum4/1
  Observer/2(x2) -> Gain1/1
  Gain1/1 -> Sum3/2
  Gain/1 -> Sum3/1
  ref/1 -> Sum/1
  Observer/1(x3) -> Sum4/2
  Observer/3(x1) -> Sum/2

== system PSO_ZVD/RBF_ZVD_m=5_m1=1/ADRC 9 ==
  ref : Inport
  x : Inport  Port=2
  Gain : Gain  Gain=Kp
  Gain1 : Gain  Gain=Kd
  Gain2 : Gain  Gain=1/b0
  Observer : Subsystem
  Sum : Sum  Inputs=|+-
  Sum3 : Sum  Inputs=|+-
  Sum4 : Sum  Inputs=|+-
  u : Outport
  wires:
  Sum4/1 -> Gain2/1
  Sum/1 -> Gain/1
  Gain2/1 -> u/1, Observer/1(u)
  x/1 -> Observer/2(x)
  Sum3/1 -> Sum4/1
  Observer/2(x2) -> Gain1/1
  Gain1/1 -> Sum3/2
  Gain/1 -> Sum3/1
  ref/1 -> Sum/1
  Observer/1(x3) -> Sum4/2
  Observer/3(x1) -> Sum/2

== system PSO_ZVD/RBF_ZVD_m=5_m1=1/PSO-ETM1 ==
  In1 : Inport
  Input : Inport  Port=2
  Input1 : Inport  Port=3
  Gain : Gain  Gain=0.25
  Gain1 : Gain  Gain=0.5
  Gain2 : Gain  Gain=0.25
  Sum : Sum  Inputs=+++
  Variable Transport Delay : VariableTransportDelay  VariableDelayType=Variable transport delay  MaximumDelay=10
  Variable Transport Delay1 : VariableTransportDelay  VariableDelayType=Variable transport delay  MaximumDelay=10
  Out1 : Outport
  wires:
  In1/1 -> Gain1/1, Gain2/1, Gain/1
  Gain1/1 -> Variable Transport Delay/1
  Variable Transport Delay/1 -> Sum/2
  Sum/1 -> Out1/1
  Gain2/1 -> Variable Transport Delay1/1
  Gain/1 -> Sum/1
  Variable Transport Delay1/1 -> Sum/3
  Input/1 -> Variable Transport Delay/2
  Input1/1 -> Variable Transport Delay1/2

== system PSO_ZVD/RBF_ZVD_m=5_m1=1/PSO-ETM2 ==
  In1 : Inport
  Input : Inport  Port=2
  Input1 : Inport  Port=3
  Gain : Gain  Gain=0.25
  Gain1 : Gain  Gain=0.5
  Gain2 : Gain  Gain=0.25
  Sum : Sum  Inputs=+++
  Variable Transport Delay : VariableTransportDelay  VariableDelayType=Variable transport delay  MaximumDelay=10
  Variable Transport Delay1 : VariableTransportDelay  VariableDelayType=Variable transport delay  MaximumDelay=10
  ref : Outport
  wires:
  In1/1 -> Gain1/1, Gain2/1, Gain/1
  Gain1/1 -> Variable Transport Delay/1
  Variable Transport Delay/1 -> Sum/2
  Sum/1 -> ref/1
  Gain2/1 -> Variable Transport Delay1/1
  Gain/1 -> Sum/1
  Variable Transport Delay1/1 -> Sum/3
  Input/1 -> Variable Transport Delay/2
  Input1/1 -> Variable Transport Delay1/2

== system PSO_ZVD/RBF_ZVD_m=5_m1=1/PSO-ETM3 ==
  In1 : Inport
  Input : Inport  Port=2
  Input1 : Inport  Port=3
  Gain : Gain  Gain=0.25
  Gain1 : Gain  Gain=0.5
  Gain2 : Gain  Gain=0.25
  Sum : Sum  Inputs=+++
  Variable Transport Delay : VariableTransportDelay  VariableDelayType=Variable transport delay  MaximumDelay=10
  Variable Transport Delay1 : VariableTransportDelay  VariableDelayType=Variable transport delay  MaximumDelay=10
  ref : Outport
  wires:
  In1/1 -> Gain1/1, Gain2/1, Gain/1
  Gain1/1 -> Variable Transport Delay/1
  Variable Transport Delay/1 -> Sum/2
  Sum/1 -> ref/1
  Gain2/1 -> Variable Transport Delay1/1
  Gain/1 -> Sum/1
  Variable Transport Delay1/1 -> Sum/3
  Input/1 -> Variable Transport Delay/2
  Input1/1 -> Variable Transport Delay1/2

== system PSO_ZVD/RBF_ZVD_m=5_m1=1/PSO-ETM4 ==
  In1 : Inport
  Input : Inport  Port=2
  Input1 : Inport  Port=3
  Gain : Gain  Gain=0.25
  Gain1 : Gain  Gain=0.5
  Gain2 : Gain  Gain=0.25
  Sum : Sum  Inputs=+++
  Variable Transport Delay : VariableTransportDelay  VariableDelayType=Variable transport delay  MaximumDelay=10
  Variable Transport Delay1 : VariableTransportDelay  VariableDelayType=Variable transport delay  MaximumDelay=10
  Out1 : Outport
  wires:
  In1/1 -> Gain1/1, Gain2/1, Gain/1
  Gain1/1 -> Variable Transport Delay/1
  Variable Transport Delay/1 -> Sum/2
  Sum/1 -> Out1/1
  Gain2/1 -> Variable Transport Delay1/1
  Gain/1 -> Sum/1
  Variable Transport Delay1/1 -> Sum/3
  Input/1 -> Variable Transport Delay/2
  Input1/1 -> Variable Transport Delay1/2

== system PSO_ZVD/RBF_ZVD_m=5_m1=1/PSO-ETM5 ==
  In1 : Inport
  Input : Inport  Port=2
  Input1 : Inport  Port=3
  Gain : Gain  Gain=0.25
  Gain1 : Gain  Gain=0.5
  Gain2 : Gain  Gain=0.25
  Sum : Sum  Inputs=+++
  Variable Transport Delay : VariableTransportDelay  VariableDelayType=Variable transport delay  MaximumDelay=10
  Variable Transport Delay1 : VariableTransportDelay  VariableDelayType=Variable transport delay  MaximumDelay=10
  Out1 : Outport
  wires:
  In1/1 -> Gain1/1, Gain2/1, Gain/1
  Gain1/1 -> Variable Transport Delay/1
  Variable Transport Delay/1 -> Sum/2
  Sum/1 -> Out1/1
  Gain2/1 -> Variable Transport Delay1/1
  Gain/1 -> Sum/1
  Variable Transport Delay1/1 -> Sum/3
  Input/1 -> Variable Transport Delay/2
  Input1/1 -> Variable Transport Delay1/2

== system PSO_ZVD/RBF_ZVD_m=5_m1=1/T-ZVD ==
  ref : Inport
  Gain : Gain  Gain=0.25
  Gain1 : Gain  Gain=0.5
  Gain2 : Gain  Gain=0.25
  Sum : Sum  Inputs=+++
  Transport Delay : TransportDelay  DelayTime=t1_ZVD_1
  Transport Delay1 : TransportDelay  DelayTime=t2_ZVD_1
  ref_AZ : Outport
  wires:
  Gain1/1 -> Transport Delay/1
  Gain/1 -> Sum/1
  Transport Delay/1 -> Sum/2
  Sum/1 -> ref_AZ/1
  ref/1 -> Gain/1, Gain2/1, Gain1/1
  Gain2/1 -> Transport Delay1/1
  Transport Delay1/1 -> Sum/3

== system PSO_ZVD/RBF_ZVD_m=5_m1=1/T-ZVD1 ==
  ref : Inport
  Gain : Gain  Gain=0.25
  Gain1 : Gain  Gain=0.5
  Gain2 : Gain  Gain=0.25
  Sum : Sum  Inputs=+++
  Transport Delay : TransportDelay  DelayTime=t1_ZVD_2
  Transport Delay1 : TransportDelay  DelayTime=t2_ZVD_2
  ref_AZ : Outport
  wires:
  Gain1/1 -> Transport Delay/1
  Gain/1 -> Sum/1
  Transport Delay/1 -> Sum/2
  Sum/1 -> ref_AZ/1
  ref/1 -> Gain/1, Gain2/1, Gain1/1
  Gain2/1 -> Transport Delay1/1
  Transport Delay1/1 -> Sum/3

== system PSO_ZVD/RBF_ZVD_m=5_m1=1/T-ZVD2 ==
  ref : Inport
  Gain : Gain  Gain=0.25
  Gain1 : Gain  Gain=0.5
  Gain2 : Gain  Gain=0.25
  Sum : Sum  Inputs=+++
  Transport Delay : TransportDelay  DelayTime=t1_ZVD_2
  Transport Delay1 : TransportDelay  DelayTime=t2_ZVD_2
  ref_AZ : Outport
  wires:
  Gain1/1 -> Transport Delay/1
  Gain/1 -> Sum/1
  Transport Delay/1 -> Sum/2
  Sum/1 -> ref_AZ/1
  ref/1 -> Gain/1, Gain2/1, Gain1/1
  Gain2/1 -> Transport Delay1/1
  Transport Delay1/1 -> Sum/3

== system PSO_ZVD/RBF_ZVD_m=5_m1=1/ZVD ==
  ZVD : Inport
  T-ZVD : Subsystem
  T-ZVD1 : Subsystem
  ref1 : Scope
  ref2 : Scope
  ref3 : Scope
  zvd : Outport
  wires:
  T-ZVD/1(ref_AZ) -> T-ZVD1/1(ref), ref2/1  "ref_ZV"
  T-ZVD1/1(ref_AZ) -> ref3/1, zvd/1  "ref_ZV"
  ZVD/1 -> T-ZVD/1(ref), ref1/1

== system PSO_ZVD/RBF_ZVD_m=5_m1=1/enhanced1 ==
  Fx : Inport
  Fl : Inport  Port=2
  Add : Sum
  Constant : Constant  Value=-(m1+m2)*g
  Constant1 : Constant  Value=mc
  Crane : MATLAB Function  TreatAsAtomicUnit=on
  Integrator{,1,3,5..7} (6 alike) : Integrator
  Integrator2 : Integrator  InitialCondition=l
  Integrator4 : Integrator  InitialCondition=10*pi/180
  Scope{1..5} (5 alike) : Scope
  x : Outport
  l : Outport  Port=2
  the1 : Outport  Port=3
  the2 : Outport  Port=4
  wires:
  Integrator5/1 -> [x6]
  Integrator2/1 -> Scope4/1, l/1, [x3]
  Integrator1/1 -> [x2]
  Integrator/1 -> x/1, [x1]
  Integrator3/1 -> [x4]
  Add/1 -> Crane/9(Fl), Scope1/1
  Integrator6/1 -> Scope2/1, the2/1, [x7]
  Integrator7/1 -> [x8]
  Crane/1(dx1) -> Integrator/1
  Crane/2(dx2) -> Integrator1/1
  Crane/3(dx3) -> Integrator2/1
  Crane/4(dx4) -> Integrator3/1
  Crane/5(dx5) -> Integrator4/1
  Crane/6(dx6) -> Integrator5/1
  Crane/7(dx7) -> Integrator6/1
  Crane/8(dx8) -> Integrator7/1
  Fx/1 -> Crane/8(Fx)
  Constant1/1 -> Crane/10(m2)
  [x2] -> Crane/1(d1x)
  [x3] -> Crane/2(l1)
  [x4] -> Crane/3(d1l1)
  [x5] -> Crane/4(the1)
  [x6] -> Crane/5(d1the1)
  [x7] -> Crane/6(the2)
  [x8] -> Crane/7(d1the2)
  Integrator4/1 -> Scope3/1, the1/1, [x5]
  Fl/1 -> Add/2
  [x1] -> Scope5/1
  Constant/1 -> Add/1

== system PSO_ZVD/RBF_ZVD_m=5_m1=1/enhanced2 ==
  Fx : Inport
  Fl : Inport  Port=2
  Add : Sum
  Constant : Constant  Value=-(m1+m2)*g
  Constant1 : Constant  Value=mc
  Crane : MATLAB Function  TreatAsAtomicUnit=on
  Integrator{,1,3,5..7} (6 alike) : Integrator
  Integrator2 : Integrator  InitialCondition=l
  Integrator4 : Integrator  InitialCondition=10*pi/180
  Scope{1..5} (5 alike) : Scope
  x : Outport
  l : Outport  Port=2
  the1 : Outport  Port=3
  the2 : Outport  Port=4
  wires:
  Integrator5/1 -> [x6]
  Integrator2/1 -> Scope4/1, l/1, [x3]
  Integrator1/1 -> [x2]
  Integrator/1 -> x/1, [x1]
  Integrator3/1 -> [x4]
  Add/1 -> Crane/9(Fl), Scope1/1
  Integrator6/1 -> Scope2/1, the2/1, [x7]
  Integrator7/1 -> [x8]
  Crane/1(dx1) -> Integrator/1
  Crane/2(dx2) -> Integrator1/1
  Crane/3(dx3) -> Integrator2/1
  Crane/4(dx4) -> Integrator3/1
  Crane/5(dx5) -> Integrator4/1
  Crane/6(dx6) -> Integrator5/1
  Crane/7(dx7) -> Integrator6/1
  Crane/8(dx8) -> Integrator7/1
  Fx/1 -> Crane/8(Fx)
  Constant1/1 -> Crane/10(m2)
  [x2] -> Crane/1(d1x)
  [x3] -> Crane/2(l1)
  [x4] -> Crane/3(d1l1)
  [x5] -> Crane/4(the1)
  [x6] -> Crane/5(d1the1)
  [x7] -> Crane/6(the2)
  [x8] -> Crane/7(d1the2)
  Integrator4/1 -> Scope3/1, the1/1, [x5]
  Fl/1 -> Add/2
  [x1] -> Scope5/1
  Constant/1 -> Add/1

== system PSO_ZVD/RBF_ZVD_m=5_m1=1/enhanced3 ==
  Fx : Inport
  Fl : Inport  Port=2
  Add : Sum
  Constant : Constant  Value=-(m1+m2)*g
  Constant1 : Constant  Value=mc
  Crane : MATLAB Function  TreatAsAtomicUnit=on
  Integrator{,1,3,5..7} (6 alike) : Integrator
  Integrator2 : Integrator  InitialCondition=l
  Integrator4 : Integrator  InitialCondition=10*pi/180
  Scope{1..5} (5 alike) : Scope
  x : Outport
  l : Outport  Port=2
  the1 : Outport  Port=3
  the2 : Outport  Port=4
  wires:
  Integrator5/1 -> [x6]
  Integrator2/1 -> Scope4/1, l/1, [x3]
  Integrator1/1 -> [x2]
  Integrator/1 -> x/1, [x1]
  Integrator3/1 -> [x4]
  Add/1 -> Crane/9(Fl), Scope1/1
  Integrator6/1 -> Scope2/1, the2/1, [x7]
  Integrator7/1 -> [x8]
  Crane/1(dx1) -> Integrator/1
  Crane/2(dx2) -> Integrator1/1
  Crane/3(dx3) -> Integrator2/1
  Crane/4(dx4) -> Integrator3/1
  Crane/5(dx5) -> Integrator4/1
  Crane/6(dx6) -> Integrator5/1
  Crane/7(dx7) -> Integrator6/1
  Crane/8(dx8) -> Integrator7/1
  Fx/1 -> Crane/8(Fx)
  Constant1/1 -> Crane/10(m2)
  [x2] -> Crane/1(d1x)
  [x3] -> Crane/2(l1)
  [x4] -> Crane/3(d1l1)
  [x5] -> Crane/4(the1)
  [x6] -> Crane/5(d1the1)
  [x7] -> Crane/6(the2)
  [x8] -> Crane/7(d1the2)
  Integrator4/1 -> Scope3/1, the1/1, [x5]
  Fl/1 -> Add/2
  [x1] -> Scope5/1
  Constant/1 -> Add/1

== system PSO_ZVD/RBF_ZVD_m=5_m1=1/enhanced4 ==
  Fx : Inport
  Fl : Inport  Port=2
  Add : Sum
  Constant : Constant  Value=-(m1+m2)*g
  Constant1 : Constant  Value=mc
  Crane : MATLAB Function  TreatAsAtomicUnit=on
  Integrator{,1,3,5..7} (6 alike) : Integrator
  Integrator2 : Integrator  InitialCondition=l
  Integrator4 : Integrator  InitialCondition=10*pi/180
  Scope{1..5} (5 alike) : Scope
  x : Outport
  l : Outport  Port=2
  the1 : Outport  Port=3
  the2 : Outport  Port=4
  wires:
  Integrator5/1 -> [x6]
  Integrator2/1 -> Scope4/1, l/1, [x3]
  Integrator1/1 -> [x2]
  Integrator/1 -> x/1, [x1]
  Integrator3/1 -> [x4]
  Add/1 -> Crane/9(Fl), Scope1/1
  Integrator6/1 -> Scope2/1, the2/1, [x7]
  Integrator7/1 -> [x8]
  Crane/1(dx1) -> Integrator/1
  Crane/2(dx2) -> Integrator1/1
  Crane/3(dx3) -> Integrator2/1
  Crane/4(dx4) -> Integrator3/1
  Crane/5(dx5) -> Integrator4/1
  Crane/6(dx6) -> Integrator5/1
  Crane/7(dx7) -> Integrator6/1
  Crane/8(dx8) -> Integrator7/1
  Fx/1 -> Crane/8(Fx)
  Constant1/1 -> Crane/10(m2)
  [x2] -> Crane/1(d1x)
  [x3] -> Crane/2(l1)
  [x4] -> Crane/3(d1l1)
  [x5] -> Crane/4(the1)
  [x6] -> Crane/5(d1the1)
  [x7] -> Crane/6(the2)
  [x8] -> Crane/7(d1the2)
  Integrator4/1 -> Scope3/1, the1/1, [x5]
  Fl/1 -> Add/2
  [x1] -> Scope5/1
  Constant/1 -> Add/1

== system PSO_ZVD/RBF_ZVD_m=5_m1=1/enhanced5 ==
  Fx : Inport
  Fl : Inport  Port=2
  Add : Sum
  Constant : Constant  Value=-(m1+m2)*g
  Constant1 : Constant  Value=mc
  Crane : MATLAB Function  TreatAsAtomicUnit=on
  Integrator{,1,3,5..7} (6 alike) : Integrator
  Integrator2 : Integrator  InitialCondition=l
  Integrator4 : Integrator  InitialCondition=10*pi/180
  Scope{1..5} (5 alike) : Scope
  x : Outport
  l : Outport  Port=2
  the1 : Outport  Port=3
  the2 : Outport  Port=4
  wires:
  Integrator5/1 -> [x6]
  Integrator2/1 -> Scope4/1, l/1, [x3]
  Integrator1/1 -> [x2]
  Integrator/1 -> x/1, [x1]
  Integrator3/1 -> [x4]
  Add/1 -> Crane/9(Fl), Scope1/1
  Integrator6/1 -> Scope2/1, the2/1, [x7]
  Integrator7/1 -> [x8]
  Crane/1(dx1) -> Integrator/1
  Crane/2(dx2) -> Integrator1/1
  Crane/3(dx3) -> Integrator2/1
  Crane/4(dx4) -> Integrator3/1
  Crane/5(dx5) -> Integrator4/1
  Crane/6(dx6) -> Integrator5/1
  Crane/7(dx7) -> Integrator6/1
  Crane/8(dx8) -> Integrator7/1
  Fx/1 -> Crane/8(Fx)
  Constant1/1 -> Crane/10(m2)
  [x2] -> Crane/1(d1x)
  [x3] -> Crane/2(l1)
  [x4] -> Crane/3(d1l1)
  [x5] -> Crane/4(the1)
  [x6] -> Crane/5(d1the1)
  [x7] -> Crane/6(the2)
  [x8] -> Crane/7(d1the2)
  Integrator4/1 -> Scope3/1, the1/1, [x5]
  Fl/1 -> Add/2
  [x1] -> Scope5/1
  Constant/1 -> Add/1

== system PSO_ZVD/RBF_ZVD_m=5_m1=1/enhanced6 ==
  Fx : Inport
  Fl : Inport  Port=2
  Add : Sum
  Constant : Constant  Value=-(m1+m2)*g
  Constant1 : Constant  Value=mc
  Crane : MATLAB Function  TreatAsAtomicUnit=on
  Integrator{,1,3,5..7} (6 alike) : Integrator
  Integrator2 : Integrator  InitialCondition=l
  Integrator4 : Integrator  InitialCondition=10*pi/180
  Scope{1..5} (5 alike) : Scope
  x : Outport
  l : Outport  Port=2
  the1 : Outport  Port=3
  the2 : Outport  Port=4
  wires:
  Integrator5/1 -> [x6]
  Integrator2/1 -> Scope4/1, l/1, [x3]
  Integrator1/1 -> [x2]
  Integrator/1 -> x/1, [x1]
  Integrator3/1 -> [x4]
  Add/1 -> Crane/9(Fl), Scope1/1
  Integrator6/1 -> Scope2/1, the2/1, [x7]
  Integrator7/1 -> [x8]
  Crane/1(dx1) -> Integrator/1
  Crane/2(dx2) -> Integrator1/1
  Crane/3(dx3) -> Integrator2/1
  Crane/4(dx4) -> Integrator3/1
  Crane/5(dx5) -> Integrator4/1
  Crane/6(dx6) -> Integrator5/1
  Crane/7(dx7) -> Integrator6/1
  Crane/8(dx8) -> Integrator7/1
  Fx/1 -> Crane/8(Fx)
  Constant1/1 -> Crane/10(m2)
  [x2] -> Crane/1(d1x)
  [x3] -> Crane/2(l1)
  [x4] -> Crane/3(d1l1)
  [x5] -> Crane/4(the1)
  [x6] -> Crane/5(d1the1)
  [x7] -> Crane/6(the2)
  [x8] -> Crane/7(d1the2)
  Integrator4/1 -> Scope3/1, the1/1, [x5]
  Fl/1 -> Add/2
  [x1] -> Scope5/1
  Constant/1 -> Add/1
